simulink model "gm_sampleModel1503_sub"  (R2023a)
settings: Solver=VariableStepAuto  StartTime=0.0  StopTime=10.0  RelTol=1e-3
libraries: hdlsllib x1
settings Model: Creator=user1  LastModifiedBy=user1
settings OptimizationCC: BlockReduction=off  ConditionallyExecuteInputs=off
settings DebuggingCC: InheritedTsInSrcMsg=none

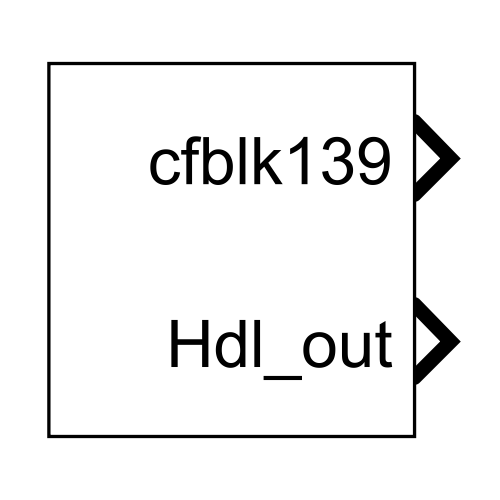
[thumbnail: Simulink's stored preview of the top-level diagram]
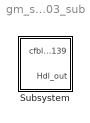
== system gm_sampleModel1503_sub ==
  Subsystem : Subsystem

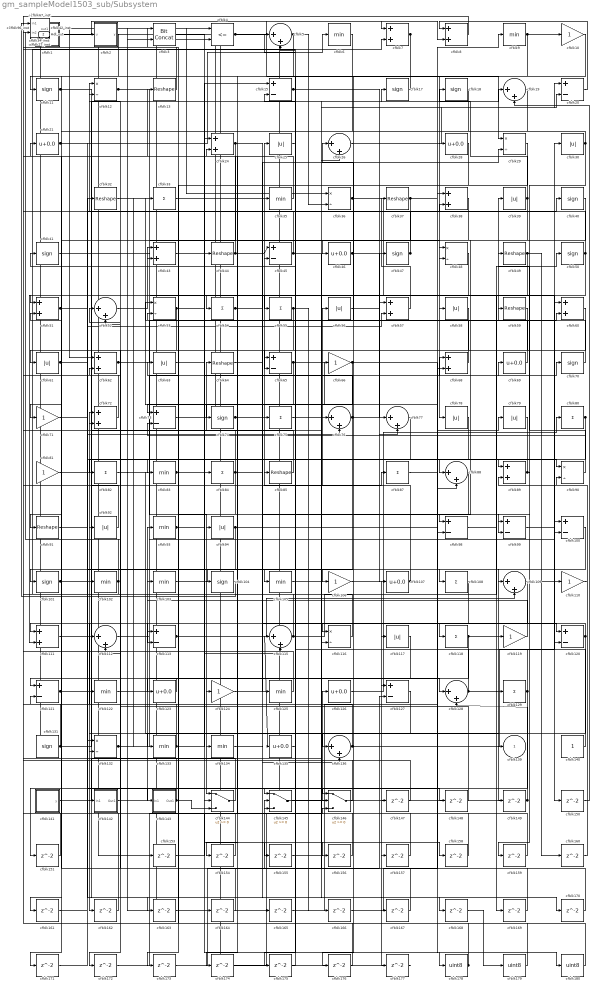
== system gm_sampleModel1503_sub/Subsystem ==
  cfblk1 : Subsystem  mask(Compare To Zero){relop=<=, OutDataTypeStr=uint8, ZeroCross=on}
      mask prompts: relop "Simulink:masks:Operator_MP"; OutDataTypeStr "Simulink:masks:OutputDataType_MP"; ZeroCross "Simulink:masks:EnableZerocrossingDetection_MP"
      mask help: Simulink:masks:CompareToZero_MD
      mask init:
      | OutDataTypeStr = 'uint8';
      | ZeroCross = 'on';
      | blkName = 'sampleModel1503_sub/Subsystem/cfblk1';
      | relop = '<=';
      | setValue = 'fixdt(0, 8)';
      mask TypeOptions relop: == | ~= | < | <= | >= | >
      mask TypeOptions OutDataTypeStr: Simulink:masks:uint8 | Simulink:masks:boolean
      mask Callback ZeroCross: sl('zeroCrossEnable', gcbh);
      mask Display: disp([relop,' 0'])
  cfblk{10,66,71,81,106,110,119,124} (8 alike) : Gain  OutDataTypeStr=uint8
  cfblk{15,20,45,65,73,98..100,113,120..121,127} (12 alike) : Sum  Inputs=+-  OutDataTypeStr=uint8
  cfblk{11,17..18,40..41,47,50,70,74,101,104,131} (12 alike) : Signum
  cfblk{6,9,35,83,93,102..103,105,122,125,133..134} (12 alike) : MinMax  OutDataTypeStr=uint8
  cfblk{21,28,46,69,107,123,126,135} (8 alike) : Bias  Bias=0.0  SaturateOnIntegerOverflow=off
  cfblk{33,54..55,75,80,82,84,87,108,118,129} (11 alike) : Sum  Inputs=+  OutDataTypeStr=uint8
  cfblk{5,19,26,52,76..77,88,109,112,115,128,136} (12 alike) : Sum  Inputs=|++  OutDataTypeStr=uint8
  cfblk{7..8,24,38,43,51,57,60,62,68,72,89,111} (13 alike) : Sum  OutDataTypeStr=uint8
  cfblk114_inst : Subsystem
  cfblk{12,29,36,48,53,90,116,132} (8 alike) : Product  Inputs=*/  OutDataTypeStr=uint8  RndMeth=Zero  SaturateOnIntegerOverflow=on
  cfblk{25,30,39,56,58,61,63,78..79,92,94,117} (12 alike) : Abs  OutDataTypeStr=uint8  SaturateOnIntegerOverflow=off
  cfblk{13,32,37,44,49,59,64,85,91} (9 alike) : Reshape
  cfblk130_inst : Subsystem
  cfblk137_inst : Subsystem
  cfblk140 : Constant  OutDataTypeStr=uint8  SampleTime=-1
  cfblk141 : Subsystem  mask(Counter Free-Running){NumBits=double(16), tsamp=double(-1)}
      mask prompts: NumBits "Simulink:masks:NumberOfBits_MP"; tsamp "Simulink:masks:SampleTime_MP"
      mask help: Simulink:masks:CounterFreeRunning_MD
  cfblk142 : Subsystem
  cfblk143 : Subsystem
  cfblk144 : Switch  OutDataTypeStr=uint8  SaturateOnIntegerOverflow=off  InputSameDT=off
  cfblk145 : Switch  OutDataTypeStr=uint8  SaturateOnIntegerOverflow=off  InputSameDT=off
  cfblk146 : Switch  OutDataTypeStr=uint8  SaturateOnIntegerOverflow=off  InputSameDT=off
  cfblk{147..151,153..177} (30 alike) : Delay  SampleTime=1
  cfblk14_inst : Subsystem
  cfblk16_inst : Subsystem
  cfblk178 : DataTypeConversion  OutDataTypeStr=uint8  SaturateOnIntegerOverflow=off  RndMeth=Floor
  cfblk179 : DataTypeConversion  OutDataTypeStr=uint8  SaturateOnIntegerOverflow=off  RndMeth=Floor
  cfblk180 : DataTypeConversion  OutDataTypeStr=uint8  SaturateOnIntegerOverflow=off  RndMeth=Floor
  cfblk2 : Subsystem  mask(Compare To Zero){relop=<=, OutDataTypeStr=uint8, ZeroCross=on}
      mask prompts: relop "Simulink:masks:Operator_MP"; OutDataTypeStr "Simulink:masks:OutputDataType_MP"; ZeroCross "Simulink:masks:EnableZerocrossingDetection_MP"
      mask help: Simulink:masks:CompareToZero_MD
      mask init:
      | OutDataTypeStr = 'uint8';
      | ZeroCross = 'on';
      | blkName = 'sampleModel1503_sub/Subsystem/cfblk2';
      | relop = '<=';
      | setValue = 'fixdt(0, 8)';
      mask TypeOptions relop: == | ~= | < | <= | >= | >
      mask TypeOptions OutDataTypeStr: Simulink:masks:uint8 | Simulink:masks:boolean
      mask Callback ZeroCross: sl('zeroCrossEnable', gcbh);
      mask Display: disp([relop,' 0'])
  cfblk22_inst : Subsystem
  cfblk23_inst : Subsystem
  cfblk27_inst : Subsystem
  cfblk3 : hdlsllib/Logic and Bit Operations/Bit Concat  numInputs=2
  cfblk34_inst : Subsystem
  cfblk4 : RelationalOperator  Operator=<=  OutDataTypeStr=boolean  InputSameDT=off
  cfblk42_inst : Subsystem
  cfblk67_inst : Subsystem
  cfblk96_inst : Subsystem
  cfblk139 : Outport  OutDataTypeStr=uint8  SampleTime=1  VectorParamsAs1DForOutWhenUnconnected=off
  Hdl_out : Outport  Port=2  OutDataTypeStr=uint8  SampleTime=1
  wires:
  cfblk1/1(y) -> cfblk7/1
  cfblk10/1 -> cfblk78/1
  cfblk100/1 -> cfblk149/1
  cfblk101/1 -> cfblk38/2, cfblk17/1
  cfblk102/1 -> cfblk7/2, cfblk114_inst/2(in2)
  cfblk103/1 -> cfblk106/1
  cfblk104/1 -> cfblk23_inst/1(in1)
  cfblk105/1 -> cfblk120/1
  cfblk106/1 -> cfblk177/1
  cfblk107/1 -> cfblk56/1, cfblk25/1
  cfblk108/1 -> cfblk162/1
  cfblk109/1 -> cfblk144/1
  cfblk11/1 -> cfblk109/1, cfblk170/1
  cfblk110/1 -> cfblk89/2
  cfblk111/1 -> cfblk72/1
  cfblk112/1 -> cfblk68/1
  cfblk113/1 -> cfblk135/1, cfblk109/2
  cfblk114_inst/1(out1) -> cfblk62/1
  cfblk115/1 -> cfblk70/1, cfblk130_inst/2(in2)
  cfblk116/1 -> cfblk52/1
  cfblk117/1 -> cfblk157/1
  cfblk118/1 -> cfblk172/1, cfblk119/1
  cfblk119/1 -> cfblk93/1
  cfblk12/1 -> cfblk46/1, cfblk134/1
  cfblk120/1 -> cfblk111/1, cfblk154/1
  cfblk121/1 -> cfblk85/1, cfblk76/1
  cfblk122/1 -> cfblk128/1
  cfblk123/1 -> cfblk121/1
  cfblk124/1 -> cfblk35/1
  cfblk125/1 -> cfblk23_inst/2(in2)
  cfblk126/1 -> cfblk80/1
  cfblk127/1 -> cfblk132/2
  cfblk128/1 -> cfblk96_inst/2(in2), cfblk100/1
  cfblk129/1 -> cfblk41/1, cfblk151/1
  cfblk13/1 -> cfblk16_inst/1(in1)
  cfblk130_inst/1(out1) -> cfblk131/1
  cfblk131/1 -> cfblk64/1, cfblk14_inst/2(in2)
  cfblk132/1 -> cfblk30/1, cfblk33/1
  cfblk133/1 -> cfblk44/1, cfblk21/1, cfblk87/1
  cfblk134/1 -> cfblk168/1
  cfblk135/1 -> cfblk45/2
  cfblk136/1 -> cfblk72/2, cfblk60/1
  cfblk137_inst/1(out1) -> cfblk36/1
  cfblk14_inst/1(out1) -> cfblk77/1
  cfblk140/1 -> cfblk102/1
  cfblk141/1(y) -> cfblk26/2
  cfblk142/1(Out1) -> cfblk103/1
  cfblk143/1(Out1) -> cfblk92/1, cfblk144/3
  cfblk144/1 -> cfblk16_inst/2(in2)
  cfblk145/1 -> cfblk126/1
  cfblk146/1 -> cfblk114_inst/1(in1)
  cfblk147/1 -> cfblk132/1
  cfblk148/1 -> cfblk52/2
  cfblk149/1 -> cfblk128/2, Hdl_out/1
  cfblk15/1 -> cfblk58/1, cfblk57/1
  cfblk150/1 -> cfblk19/2
  cfblk151/1 -> cfblk22_inst/2(in2)
  cfblk153/1 -> cfblk145/2
  cfblk154/1 -> cfblk137_inst/2(in2)
  cfblk155/1 -> cfblk60/2
  cfblk156/1 -> cfblk96_inst/1(in1)
  cfblk157/1 -> cfblk62/2
  cfblk158/1 -> cfblk24/2
  cfblk159/1 -> cfblk51/2
  cfblk16_inst/1(out1) -> cfblk75/1
  cfblk160/1 -> cfblk90/2
  cfblk161/1 -> cfblk57/2
  cfblk162/1 -> cfblk67_inst/2(in2)
  cfblk163/1 -> cfblk127/2
  cfblk164/1 -> cfblk112/2
  cfblk165/1 -> cfblk68/2
  cfblk166/1 -> cfblk38/1
  cfblk167/1 -> cfblk43/1
  cfblk168/1 -> cfblk179/1
  cfblk169/1 -> cfblk121/2
  cfblk17/1 -> cfblk11/1
  cfblk170/1 -> cfblk145/3
  cfblk171/1 -> cfblk76/2
  cfblk172/1 -> cfblk146/3
  cfblk173/1 -> cfblk146/2
  cfblk174/1 -> cfblk116/2
  cfblk175/1 -> cfblk15/2
  cfblk176/1 -> cfblk53/2
  cfblk177/1 -> cfblk1/1(u)
  cfblk178/1 -> cfblk5/2, cfblk27_inst/1(in1)
  cfblk179/1 -> cfblk3/1
  cfblk18/1 -> cfblk91/1
  cfblk180/1 -> cfblk3/2
  cfblk19/1 -> cfblk146/1
  cfblk2/1(y) -> cfblk101/1
  cfblk20/1 -> cfblk8/1
  cfblk21/1 -> cfblk112/1, cfblk6/1
  cfblk22_inst/1(out1) -> cfblk137_inst/1(in1)
  cfblk23_inst/1(out1) -> cfblk4/2
  cfblk24/1 -> cfblk51/1, cfblk117/1, cfblk48/2
  cfblk25/1 -> cfblk105/1
  cfblk26/1 -> cfblk20/2
  cfblk27_inst/1(out1) -> cfblk165/1, cfblk164/1, cfblk2/1(u)
  cfblk28/1 -> cfblk133/1
  cfblk29/1 -> cfblk73/1
  cfblk3/1 -> cfblk178/1
  cfblk30/1 -> cfblk99/2, cfblk28/1
  cfblk32/1 -> cfblk77/2
  cfblk33/1 -> cfblk29/2
  cfblk34_inst/1(out1) -> cfblk42_inst/1(in1), cfblk4/1
  cfblk35/1 -> cfblk13/1
  cfblk36/1 -> cfblk120/2, cfblk129/1
  cfblk37/1 -> cfblk176/1, cfblk9/1
  cfblk38/1 -> cfblk55/1
  cfblk39/1 -> cfblk98/1, cfblk18/1
  cfblk4/1 -> cfblk8/2, cfblk29/1
  cfblk40/1 -> cfblk54/1
  cfblk41/1 -> cfblk100/2
  cfblk42_inst/1(out1) -> cfblk153/1
  cfblk43/1 -> cfblk127/1
  cfblk44/1 -> cfblk45/1, cfblk130_inst/1(in1), cfblk48/1
  cfblk45/1 -> cfblk167/1, cfblk12/1
  cfblk46/1 -> cfblk107/1, cfblk169/1
  cfblk47/1 -> cfblk5/1, cfblk14_inst/1(in1)
  cfblk48/1 -> cfblk94/1
  cfblk49/1 -> cfblk161/1, cfblk160/1, cfblk110/1
  cfblk5/1 -> cfblk61/1, cfblk36/2
  cfblk50/1 -> cfblk34_inst/2(in2), cfblk34_inst/1(in1), cfblk111/2
  cfblk51/1 -> cfblk40/1, cfblk90/1
  cfblk52/1 -> cfblk43/2
  cfblk53/1 -> cfblk15/1, cfblk71/1
  cfblk54/1 -> cfblk115/1, cfblk158/1
  cfblk55/1 -> cfblk65/2, cfblk166/1
  cfblk56/1 -> cfblk89/1
  cfblk57/1 -> cfblk37/1
  cfblk58/1 -> cfblk142/1(In1)
  cfblk59/1 -> cfblk83/1
  cfblk6/1 -> cfblk65/1
  cfblk60/1 -> cfblk143/1(In1)
  cfblk61/1 -> cfblk163/1, cfblk108/1
  cfblk62/1 -> cfblk74/1, cfblk47/1
  cfblk63/1 -> cfblk155/1
  cfblk64/1 -> cfblk125/1
  cfblk65/1 -> cfblk98/2, cfblk113/2
  cfblk66/1 -> cfblk88/2, cfblk123/1
  cfblk67_inst/1(out1) -> cfblk84/1
  cfblk68/1 -> cfblk53/1
  cfblk69/1 -> cfblk26/1
  cfblk7/1 -> cfblk145/1, cfblk136/1
  cfblk70/1 -> cfblk39/1
  cfblk71/1 -> cfblk148/1
  cfblk72/1 -> cfblk42_inst/2(in2)
  cfblk73/1 -> cfblk147/1
  cfblk74/1 -> cfblk99/1, cfblk136/2
  cfblk75/1 -> cfblk20/1
  cfblk76/1 -> cfblk69/1, cfblk59/1, cfblk24/1, cfblk113/1
  cfblk77/1 -> cfblk144/2
  cfblk78/1 -> cfblk122/1
  cfblk79/1 -> cfblk104/1
  cfblk8/1 -> cfblk22_inst/1(in1)
  cfblk80/1 -> cfblk73/2, cfblk116/1
  cfblk81/1 -> cfblk19/1
  cfblk82/1 -> cfblk139/1
  cfblk83/1 -> cfblk88/1, cfblk156/1
  cfblk84/1 -> cfblk27_inst/2(in2), cfblk173/1, cfblk12/2, cfblk118/1
  cfblk85/1 -> cfblk63/1
  cfblk87/1 -> cfblk79/1
  cfblk88/1 -> cfblk124/1
  cfblk89/1 -> cfblk159/1, cfblk82/1
  cfblk9/1 -> cfblk175/1, cfblk174/1, cfblk10/1
  cfblk90/1 -> cfblk49/1
  cfblk91/1 -> cfblk32/1
  cfblk92/1 -> cfblk67_inst/1(in1)
  cfblk93/1 -> cfblk115/2, cfblk66/1
  cfblk94/1 -> cfblk180/1, cfblk171/1
  cfblk96_inst/1(out1) -> cfblk81/1
  cfblk98/1 -> cfblk50/1
  cfblk99/1 -> cfblk150/1

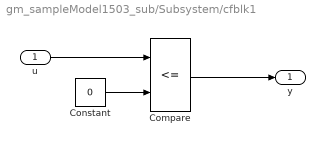
== system gm_sampleModel1503_sub/Subsystem/cfblk1 ==
  u : Inport  OutDataTypeStr=uint8  SampleTime=1
  Compare : RelationalOperator  Operator=<=  OutDataTypeStr=fixdt(0, 8)
  Constant : Constant  DisableCoverage=on  Value=0  OutDataTypeStr=Inherit: Inherit via back propagation  SampleTime=-1  PreserveConstantTs=on
  y : Outport  SampleTime=1
  wires:
  u/1 -> Compare/1
  Compare/1 -> y/1
  Constant/1 -> Compare/2

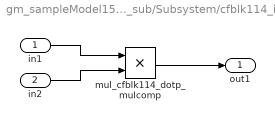
== system gm_sampleModel1503_sub/Subsystem/cfblk114_inst ==
  in1 : Inport  OutDataTypeStr=uint8  SampleTime=1
  in2 : Inport  Port=2  OutDataTypeStr=uint8  SampleTime=1
  mul_cfblk114_dotp_mulcomp : Product  Inputs=**  OutDataTypeStr=uint8  SampleTime=1
  out1 : Outport  OutDataTypeStr=uint8  SampleTime=1
  wires:
  in1/1 -> mul_cfblk114_dotp_mulcomp/1
  in2/1 -> mul_cfblk114_dotp_mulcomp/2
  mul_cfblk114_dotp_mulcomp/1 -> out1/1

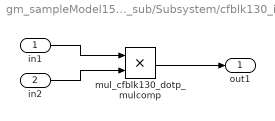
== system gm_sampleModel1503_sub/Subsystem/cfblk130_inst ==
  in1 : Inport  OutDataTypeStr=uint8  SampleTime=1
  in2 : Inport  Port=2  OutDataTypeStr=uint8  SampleTime=1
  mul_cfblk130_dotp_mulcomp : Product  Inputs=**  OutDataTypeStr=uint8  SampleTime=1
  out1 : Outport  OutDataTypeStr=uint8  SampleTime=1
  wires:
  in1/1 -> mul_cfblk130_dotp_mulcomp/1
  in2/1 -> mul_cfblk130_dotp_mulcomp/2
  mul_cfblk130_dotp_mulcomp/1 -> out1/1

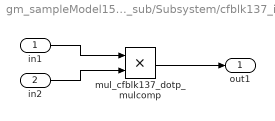
== system gm_sampleModel1503_sub/Subsystem/cfblk137_inst ==
  in1 : Inport  OutDataTypeStr=uint8  SampleTime=1
  in2 : Inport  Port=2  OutDataTypeStr=uint8  SampleTime=1
  mul_cfblk137_dotp_mulcomp : Product  Inputs=**  OutDataTypeStr=uint8  SampleTime=1
  out1 : Outport  OutDataTypeStr=uint8  SampleTime=1
  wires:
  in1/1 -> mul_cfblk137_dotp_mulcomp/1
  in2/1 -> mul_cfblk137_dotp_mulcomp/2
  mul_cfblk137_dotp_mulcomp/1 -> out1/1

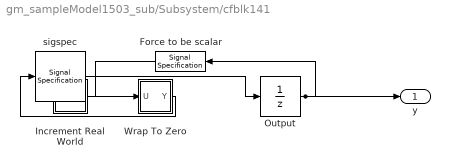
== system gm_sampleModel1503_sub/Subsystem/cfblk141 ==
  Force to be scalar : SignalSpecification  DisableCoverage=on  Dimensions=1
  Increment Real World : Subsystem  mask(Real World Value Increment){}
      mask help: Simulink:masks:RealWorldValueIncrement_MD
      mask Display: disp('V++')
  Output : UnitDelay  InitialCondition=0.0  SampleTime=tsamp  HasFrameUpgradeWarning=on
  Wrap To Zero : Subsystem  mask(Wrap To Zero){Threshold=double(65535)}
      mask prompts: Threshold "Simulink:masks:Threshold_MP"
      mask help: Simulink:masks:WrapToZero_MD
  sigspec : SignalSpecification  OutDataTypeStr=uint16  Dimensions=1
  y : Outport  SampleTime=1
  wires:
  Force to be scalar/1 -> Increment Real World/1(u)
  Increment Real World/1(y) -> Wrap To Zero/1(U)
  Output/1 -> Force to be scalar/1, y/1
  Wrap To Zero/1(Y) -> sigspec/1
  sigspec/1 -> Output/1

== system gm_sampleModel1503_sub/Subsystem/cfblk142 ==
  In1 : Inport  OutDataTypeStr=uint8  PortDimensions=1  SampleTime=1
  Out1 : Outport  SampleTime=1
  wires:
  In1/1 -> Out1/1

== system gm_sampleModel1503_sub/Subsystem/cfblk143 ==
  In1 : Inport  OutDataTypeStr=uint8  PortDimensions=1  SampleTime=1
  Out1 : Outport  SampleTime=1
  wires:
  In1/1 -> Out1/1

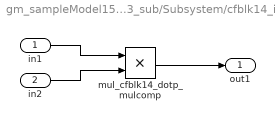
== system gm_sampleModel1503_sub/Subsystem/cfblk14_inst ==
  in1 : Inport  OutDataTypeStr=uint8  SampleTime=1
  in2 : Inport  Port=2  OutDataTypeStr=uint8  SampleTime=1
  mul_cfblk14_dotp_mulcomp : Product  Inputs=**  OutDataTypeStr=uint8  SampleTime=1
  out1 : Outport  OutDataTypeStr=uint8  SampleTime=1
  wires:
  in1/1 -> mul_cfblk14_dotp_mulcomp/1
  in2/1 -> mul_cfblk14_dotp_mulcomp/2
  mul_cfblk14_dotp_mulcomp/1 -> out1/1

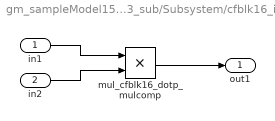
== system gm_sampleModel1503_sub/Subsystem/cfblk16_inst ==
  in1 : Inport  OutDataTypeStr=uint8  SampleTime=1
  in2 : Inport  Port=2  OutDataTypeStr=uint8  SampleTime=1
  mul_cfblk16_dotp_mulcomp : Product  Inputs=**  OutDataTypeStr=uint8  SampleTime=1
  out1 : Outport  OutDataTypeStr=uint8  SampleTime=1
  wires:
  in1/1 -> mul_cfblk16_dotp_mulcomp/1
  in2/1 -> mul_cfblk16_dotp_mulcomp/2
  mul_cfblk16_dotp_mulcomp/1 -> out1/1

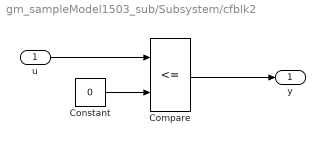
== system gm_sampleModel1503_sub/Subsystem/cfblk2 ==
  u : Inport  OutDataTypeStr=uint8  SampleTime=1
  Compare : RelationalOperator  Operator=<=  OutDataTypeStr=fixdt(0, 8)
  Constant : Constant  DisableCoverage=on  Value=0  OutDataTypeStr=Inherit: Inherit via back propagation  SampleTime=-1  PreserveConstantTs=on
  y : Outport  SampleTime=1
  wires:
  u/1 -> Compare/1
  Compare/1 -> y/1
  Constant/1 -> Compare/2

== system gm_sampleModel1503_sub/Subsystem/cfblk22_inst ==
  in1 : Inport  OutDataTypeStr=uint8  SampleTime=1
  in2 : Inport  Port=2  OutDataTypeStr=uint8  SampleTime=1
  mul_cfblk22_dotp_mulcomp : Product  Inputs=**  OutDataTypeStr=uint8  SampleTime=1
  out1 : Outport  OutDataTypeStr=uint8  SampleTime=1
  wires:
  in1/1 -> mul_cfblk22_dotp_mulcomp/1
  in2/1 -> mul_cfblk22_dotp_mulcomp/2
  mul_cfblk22_dotp_mulcomp/1 -> out1/1

== system gm_sampleModel1503_sub/Subsystem/cfblk23_inst ==
  in1 : Inport  OutDataTypeStr=uint8  SampleTime=1
  in2 : Inport  Port=2  OutDataTypeStr=uint8  SampleTime=1
  mul_cfblk23_dotp_mulcomp : Product  Inputs=**  OutDataTypeStr=uint8  SampleTime=1
  out1 : Outport  OutDataTypeStr=uint8  SampleTime=1
  wires:
  in1/1 -> mul_cfblk23_dotp_mulcomp/1
  in2/1 -> mul_cfblk23_dotp_mulcomp/2
  mul_cfblk23_dotp_mulcomp/1 -> out1/1

== system gm_sampleModel1503_sub/Subsystem/cfblk27_inst ==
  in1 : Inport  OutDataTypeStr=uint8  SampleTime=1
  in2 : Inport  Port=2  OutDataTypeStr=uint8  SampleTime=1
  mul_cfblk27_dotp_mulcomp : Product  Inputs=**  OutDataTypeStr=uint8  SampleTime=1
  out1 : Outport  OutDataTypeStr=uint8  SampleTime=1
  wires:
  in1/1 -> mul_cfblk27_dotp_mulcomp/1
  in2/1 -> mul_cfblk27_dotp_mulcomp/2
  mul_cfblk27_dotp_mulcomp/1 -> out1/1

== system gm_sampleModel1503_sub/Subsystem/cfblk34_inst ==
  in1 : Inport  OutDataTypeStr=uint8  SampleTime=1
  in2 : Inport  Port=2  OutDataTypeStr=uint8  SampleTime=1
  mul_cfblk34_dotp_mulcomp : Product  Inputs=**  OutDataTypeStr=uint8  SampleTime=1
  out1 : Outport  OutDataTypeStr=uint8  SampleTime=1
  wires:
  in1/1 -> mul_cfblk34_dotp_mulcomp/1
  in2/1 -> mul_cfblk34_dotp_mulcomp/2
  mul_cfblk34_dotp_mulcomp/1 -> out1/1

== system gm_sampleModel1503_sub/Subsystem/cfblk42_inst ==
  in1 : Inport  OutDataTypeStr=uint8  SampleTime=1
  in2 : Inport  Port=2  OutDataTypeStr=uint8  SampleTime=1
  mul_cfblk42_dotp_mulcomp : Product  Inputs=**  OutDataTypeStr=uint8  SampleTime=1
  out1 : Outport  OutDataTypeStr=uint8  SampleTime=1
  wires:
  in1/1 -> mul_cfblk42_dotp_mulcomp/1
  in2/1 -> mul_cfblk42_dotp_mulcomp/2
  mul_cfblk42_dotp_mulcomp/1 -> out1/1

== system gm_sampleModel1503_sub/Subsystem/cfblk67_inst ==
  in1 : Inport  OutDataTypeStr=uint8  SampleTime=1
  in2 : Inport  Port=2  OutDataTypeStr=uint8  SampleTime=1
  mul_cfblk67_dotp_mulcomp : Product  Inputs=**  OutDataTypeStr=uint8  SampleTime=1
  out1 : Outport  OutDataTypeStr=uint8  SampleTime=1
  wires:
  in1/1 -> mul_cfblk67_dotp_mulcomp/1
  in2/1 -> mul_cfblk67_dotp_mulcomp/2
  mul_cfblk67_dotp_mulcomp/1 -> out1/1

== system gm_sampleModel1503_sub/Subsystem/cfblk96_inst ==
  in1 : Inport  OutDataTypeStr=uint8  SampleTime=1
  in2 : Inport  Port=2  OutDataTypeStr=uint8  SampleTime=1
  mul_cfblk96_dotp_mulcomp : Product  Inputs=**  OutDataTypeStr=uint8  SampleTime=1
  out1 : Outport  OutDataTypeStr=uint8  SampleTime=1
  wires:
  in1/1 -> mul_cfblk96_dotp_mulcomp/1
  in2/1 -> mul_cfblk96_dotp_mulcomp/2
  mul_cfblk96_dotp_mulcomp/1 -> out1/1

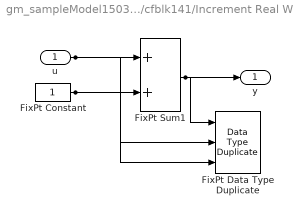
== system gm_sampleModel1503_sub/Subsystem/cfblk141/Increment Real World ==
  u : Inport  OutDataTypeStr=uint16  SampleTime=1
  FixPt Constant : Constant  DisableCoverage=on  OutDataTypeStr=Inherit: Inherit via back propagation  SampleTime=-1
  FixPt Data Type Duplicate : DataTypeDuplicate  DisableCoverage=on  NumInputPorts=3
  FixPt Sum1 : Sum  InputSameDT=on  OutDataTypeStr=Inherit: Inherit via back propagation  LockScale=on
  y : Outport  SampleTime=1
  wires:
  u/1 -> FixPt Sum1/1, FixPt Data Type Duplicate/2
  FixPt Constant/1 -> FixPt Sum1/2, FixPt Data Type Duplicate/3
  FixPt Sum1/1 -> FixPt Data Type Duplicate/1, y/1

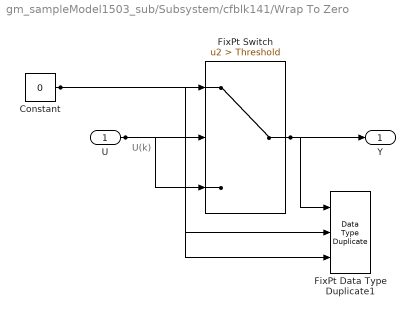
== system gm_sampleModel1503_sub/Subsystem/cfblk141/Wrap To Zero ==
  note: U(k)
  U : Inport  OutDataTypeStr=uint16  SampleTime=1
  Constant : Constant  DisableCoverage=on  Value=0  OutDataTypeStr=Inherit: Inherit via back propagation  SampleTime=-1
  FixPt Data Type Duplicate1 : DataTypeDuplicate  DisableCoverage=on  NumInputPorts=3
  FixPt Switch : Switch  Criteria=u2 > Threshold  Threshold=Threshold  OutDataTypeStr=Inherit: Inherit via back propagation  ZeroCross=off  SaturateOnIntegerOverflow=off  InputSameDT=off
  Y : Outport  SampleTime=1
  wires:
  U/1 -> FixPt Switch/3, FixPt Switch/2, FixPt Data Type Duplicate1/2
  Constant/1 -> FixPt Switch/1, FixPt Data Type Duplicate1/3
  FixPt Switch/1 -> FixPt Data Type Duplicate1/1, Y/1
